simulink model "balancingController_QP"  (Simulink 8.3)
settings: Solver=FixedStepDiscrete  StartTime=0.0  StopTime=inf  FixedStep=Ts  RelTol=1e-3
InitFcn:
  | initBalancingController;
values from neighbouring files (symbols this model uses):
  Gains = block.InputPort(14).Data    [controllerQP.m]    (also in initBalancingController.m = [  120    0   1  1]; initBalancingControllerWithNonLinearImpedances.m = [  70    0   0  4])
  Impedances = block.InputPort(15).Data    [controllerQP.m]    (also in initBalancingController.m = [kImpTorso,kImpArms,kImpArms,kImpLegs,kImpLegs])
undefined symbols (not defined in the file or in its folder): DiscIntNeverNeededParam
undefined symbols (not defined in the file): localName, robotName
libraries: WBCLibrary x18, simulink x2, dspsigops x2
settings Model: Creator=daniele  LastModifiedBy=talha
settings DataIOCC: SignalLoggingSaveFormat=Dataset
settings OptimizationCC: ExpressionDepthLimit=2147483647
settings DebuggingCC: FcnCallInpInsideContextMsg=EnableAllAsWarning
settings SFSimCC: SimParseCustomCode=off

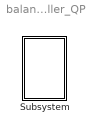
== system balancingController_QP ==
  Subsystem : Subsystem  mask{robotName=robotName, Ts=0.01, localName=localName}
      mask prompts: robotName "robot name"; localName "module name"

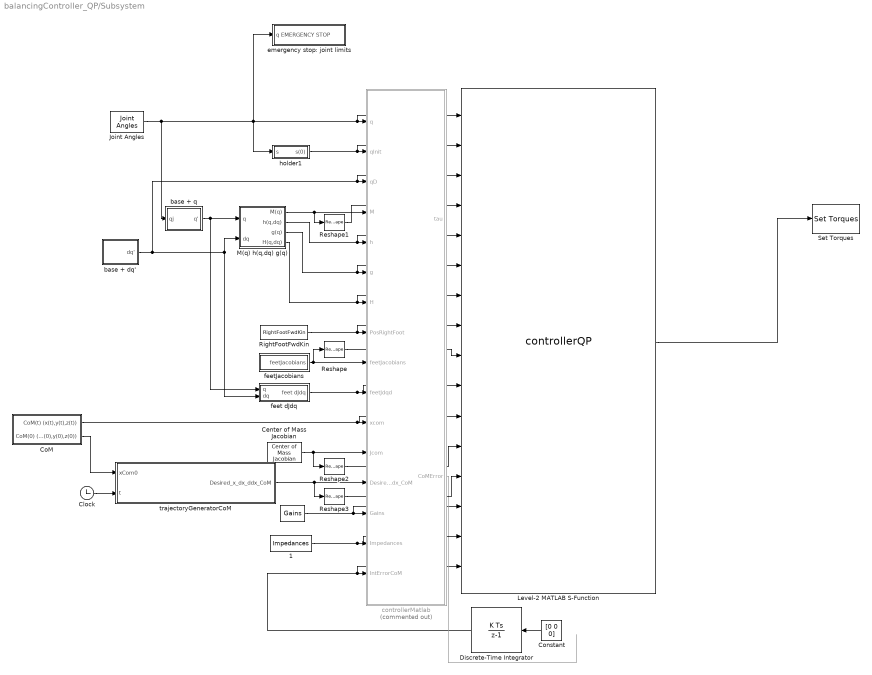
== system balancingController_QP/Subsystem ==
  "    " : Constant  Value=Gains
  "    1" : Constant  Value=Impedances
  Center of Mass Jacobian : WBCLibrary/wholeBodyModel/Jacobians/Center of Mass Jacobian  robotName=robotName  localName=localName
  Clock : Clock
  "CoM " : Subsystem
  Constant : Constant  Value=[0 0 0]
  Discrete-Time Integrator : DiscreteIntegrator  InitialCondition=[0 0 0]  SampleTime=Ts  ICPrevOutput=DiscIntNeverNeededParam  ICPrevScaledInput=DiscIntNeverNeededParam
  Joint Angles : WBCLibrary/wholeBodyStates/Joint Angles  robotName=robotName  localName=localName
  Level-2 MATLAB S-Function : M-S-Function  FunctionName=controllerQP
  M(q) h(q,dq) g(q) : Subsystem
  Reshape{,1..3} (4 alike) : Reshape
  RightFootFwdKin : WBCLibrary/wholeBodyModel/Forward Kinematics/RightFootFwdKin  robotName=robotName  localName=localName
  Set Torques : WBCLibrary/wholeBodyActuators/Set Torques  val=6  robotName=robotName  localName=localName
  base + dq' : Subsystem
  base + q : Subsystem
  controllerMatlab : MATLAB Function  Commented=on  TreatAsAtomicUnit=on
  emergency stop: joint limits : Subsystem
  feet dJdq : Subsystem
  feetJacobians : Subsystem
  holder1 : Subsystem
  trajectoryGeneratorCoM : MATLAB Function  TreatAsAtomicUnit=on
  wires:
  "    "/1 -> controllerMatlab/14(Gains), Level-2 MATLAB S-Function/14
  trajectoryGeneratorCoM/1(Desired_x_dx_ddx_CoM) -> controllerMatlab/13(Desired_x_dx_ddx_CoM), Reshape3/1
  Clock/1 -> trajectoryGeneratorCoM/2(t)
  "CoM "/2(CoM(0) (x(0),y(0),z(0))) -> trajectoryGeneratorCoM/1(xCom0)
  RightFootFwdKin/1 -> Level-2 MATLAB S-Function/8, controllerMatlab/8(PosRightFoot)
  Discrete-Time Integrator/1 -> Level-2 MATLAB S-Function/16, controllerMatlab/16(IntErrorCoM)
  base + q/1(q') -> feet dJdq/1(q), M(q) h(q,dq) g(q)/1(q)
  Joint Angles/1 -> base + q/1(qj), Level-2 MATLAB S-Function/1, controllerMatlab/1(q), emergency stop: joint limits/1(q EMERGENCY STOP), holder1/1(s)
  controllerMatlab/2(CoMError) -> ?
  "    1"/1 -> Level-2 MATLAB S-Function/15, controllerMatlab/15(Impedances)
  M(q) h(q,dq) g(q)/3(g(q)) -> Level-2 MATLAB S-Function/6, controllerMatlab/6(g)
  M(q) h(q,dq) g(q)/4(H(q,dq)) -> Level-2 MATLAB S-Function/7, controllerMatlab/7(H)
  Center of Mass Jacobian/1 -> controllerMatlab/12(Jcom), Reshape2/1
  feetJacobians/1(feetJacobians) -> controllerMatlab/9(feetJacobians), Reshape/1
  feet dJdq/1(feet dJdq) -> Level-2 MATLAB S-Function/10, controllerMatlab/10(feetJdqd)
  holder1/1(s(0)) -> Level-2 MATLAB S-Function/2, controllerMatlab/2(qInit)
  "CoM "/1(CoM(t) (x(t),y(t),z(t))) -> controllerMatlab/11(xcom), Level-2 MATLAB S-Function/11
  base + dq'/1(dq') -> Level-2 MATLAB S-Function/3, controllerMatlab/3(qD), feet dJdq/2(dq), M(q) h(q,dq) g(q)/2(dq)
  M(q) h(q,dq) g(q)/1(M(q)) -> controllerMatlab/4(M), Reshape1/1
  M(q) h(q,dq) g(q)/2(h(q,dq)) -> Level-2 MATLAB S-Function/5, controllerMatlab/5(h)
  Reshape1/1 -> Level-2 MATLAB S-Function/4
  Reshape/1 -> Level-2 MATLAB S-Function/9
  Reshape2/1 -> Level-2 MATLAB S-Function/12
  Reshape3/1 -> Level-2 MATLAB S-Function/13
  Level-2 MATLAB S-Function/1 -> Set Torques/1
  Constant/1 -> Discrete-Time Integrator/1

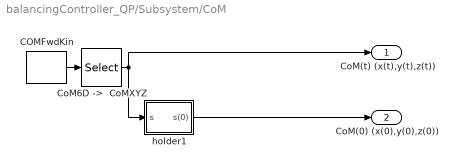
== system balancingController_QP/Subsystem/CoM  ==
  "COMFwdKin " : WBCLibrary/wholeBodyModel/Forward Kinematics/COMFwdKin   robotName=robotName  localName=localName
  "CoM6D ->  CoMXYZ" : Selector  InputPortWidth=7  Indices=[1 2 3]
  holder1 : Subsystem
  CoM(t) (x(t),y(t),z(t)) : Outport
  CoM(0) (x(0),y(0),z(0)) : Outport  Port=2
  wires:
  "COMFwdKin "/1 -> "CoM6D ->  CoMXYZ"/1
  "CoM6D ->  CoMXYZ"/1 -> holder1/1(s), CoM(t) (x(t),y(t),z(t))/1
  holder1/1(s(0)) -> CoM(0) (x(0),y(0),z(0))/1

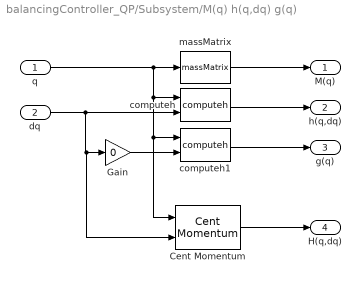
== system balancingController_QP/Subsystem/M(q) h(q,dq) g(q) ==
  q : Inport
  dq : Inport  Port=2
  Cent Momentum : WBCLibrary/wholeBodyModel/Dynamics/Cent Momentum  robotName=robotName  localName=localName
  Gain : Gain  Gain=0
  computeh : WBCLibrary/wholeBodyModel/Dynamics/computeh  val=7  robotname=robotName  localname=localName
  computeh1 : WBCLibrary/wholeBodyModel/Dynamics/computeh  val=7  robotname=robotName  localname=localName
  massMatrix : WBCLibrary/wholeBodyModel/Dynamics/massMatrix  val=8  robotname=robotName  localname=localName
  M(q) : Outport
  h(q,dq) : Outport  Port=2
  g(q) : Outport  Port=3
  H(q,dq) : Outport  Port=4
  wires:
  Gain/1 -> computeh1/2
  computeh1/1 -> g(q)/1
  computeh/1 -> h(q,dq)/1
  massMatrix/1 -> M(q)/1
  q/1 -> Cent Momentum/1, computeh1/1, computeh/1, massMatrix/1
  dq/1 -> Cent Momentum/2, Gain/1, computeh/2
  Cent Momentum/1 -> H(q,dq)/1

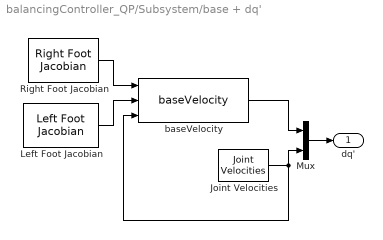
== system balancingController_QP/Subsystem/base + dq' ==
  Joint Velocities : WBCLibrary/wholeBodyStates/Joint Velocities  robotName=robotName  localName=localName
  Left Foot Jacobian : WBCLibrary/wholeBodyModel/Jacobians/Left Foot Jacobian  robotName=robotName  localName=localName
  Mux : Mux  Inputs=2
  Right Foot Jacobian : WBCLibrary/wholeBodyModel/Jacobians/Right Foot Jacobian  robotName=robotName  localName=localName
  baseVelocity : WBCLibrary/Utilities/baseVelocity
  dq' : Outport
  wires:
  Left Foot Jacobian/1 -> baseVelocity/2
  Right Foot Jacobian/1 -> baseVelocity/1
  baseVelocity/1 -> Mux/1
  Joint Velocities/1 -> baseVelocity/3, Mux/2
  Mux/1 -> dq'/1

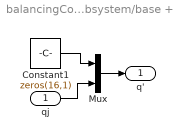
== system balancingController_QP/Subsystem/base + q ==
  qj : Inport
  Constant1 : Constant  Value=zeros(16,1)
  Mux : Mux  Inputs=2
  q' : Outport
  wires:
  Mux/1 -> q'/1
  qj/1 -> Mux/2
  Constant1/1 -> Mux/1

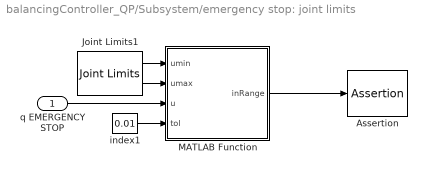
== system balancingController_QP/Subsystem/emergency stop: joint limits ==
  q EMERGENCY STOP : Inport
  Assertion : Assertion
  Joint Limits1 : WBCLibrary/wholeBodyModel/Joint Limits  robotName=robotName  localName=localName
  MATLAB Function : MATLAB Function  TreatAsAtomicUnit=on
  index1 : Constant  Value=0.01  VectorParams1D=off
  wires:
  Joint Limits1/1 -> MATLAB Function/1(umin)
  Joint Limits1/2 -> MATLAB Function/2(umax)
  index1/1 -> MATLAB Function/4(tol)
  q EMERGENCY STOP/1 -> MATLAB Function/3(u)
  MATLAB Function/1(inRange) -> Assertion/1

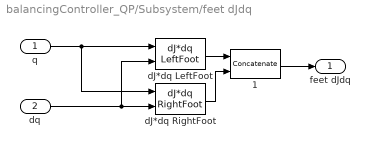
== system balancingController_QP/Subsystem/feet dJdq ==
  q : Inport
  dq : Inport  Port=2
  " 1" : Concatenate  Mode=Multidimensional array
  dJ*dq LeftFoot : WBCLibrary/wholeBodyModel/Dynamics/dJ*dq LeftFoot  val=9  robotName=robotName  localName=localName
  dJ*dq RightFoot : WBCLibrary/wholeBodyModel/Dynamics/dJ*dq RightFoot  val=9  robotName=robotName  localName=localName
  feet dJdq : Outport
  wires:
  dJ*dq LeftFoot/1 -> " 1"/1
  dJ*dq RightFoot/1 -> " 1"/2
  " 1"/1 -> feet dJdq/1
  q/1 -> dJ*dq RightFoot/1, dJ*dq LeftFoot/1
  dq/1 -> dJ*dq LeftFoot/2, dJ*dq RightFoot/2

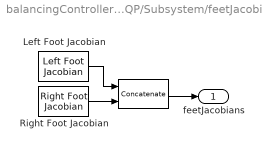
== system balancingController_QP/Subsystem/feetJacobians ==
  " " : Concatenate  Mode=Multidimensional array
  Left Foot Jacobian : WBCLibrary/wholeBodyModel/Jacobians/Left Foot Jacobian  robotName=robotName  localName=localName
  Right Foot Jacobian : WBCLibrary/wholeBodyModel/Jacobians/Right Foot Jacobian  robotName=robotName  localName=localName
  feetJacobians : Outport
  wires:
  Left Foot Jacobian/1 -> " "/1
  Right Foot Jacobian/1 -> " "/2
  " "/1 -> feetJacobians/1

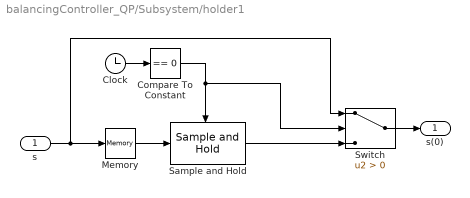
== system balancingController_QP/Subsystem/holder1 ==
  s : Inport
  Clock : Clock
  Compare To Constant : simulink/Logic and Bit Operations/Compare To Constant  relop===  const=0  OutDataTypeStr=boolean
  Memory : Memory
  Sample and Hold : dspsigops/Sample and Hold  trig=Falling edge  initCond=0  latchinput=off
  Switch : Switch  Criteria=u2 > Threshold
  s(0) : Outport
  wires:
  s/1 -> Switch/1, Memory/1
  Clock/1 -> Compare To Constant/1
  Compare To Constant/1 -> Sample and Hold/Trigger, Switch/2
  Sample and Hold/1 -> Switch/3
  Switch/1 -> s(0)/1
  Memory/1 -> Sample and Hold/1

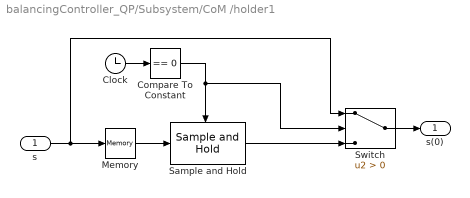
== system balancingController_QP/Subsystem/CoM /holder1 ==
  s : Inport
  Clock : Clock
  Compare To Constant : simulink/Logic and Bit Operations/Compare To Constant  relop===  const=0  OutDataTypeStr=boolean
  Memory : Memory
  Sample and Hold : dspsigops/Sample and Hold  trig=Falling edge  initCond=0  latchinput=off
  Switch : Switch  Criteria=u2 > Threshold
  s(0) : Outport
  wires:
  s/1 -> Switch/1, Memory/1
  Clock/1 -> Compare To Constant/1
  Compare To Constant/1 -> Sample and Hold/Trigger, Switch/2
  Sample and Hold/1 -> Switch/3
  Switch/1 -> s(0)/1
  Memory/1 -> Sample and Hold/1

== matlab function Subsystem/trajectoryGeneratorCoM ==
  data: Desired_x_dx_ddx_CoM output double; xCom0 input double; t input double
function Desired_x_dx_ddx_CoM = fcn(xCom0,t)
%#codegen

e3 = [0;1;0];
A = 0.0;
f = 0.05;

xcomDes    = xCom0 + A*sin(2*pi*f*t)*e3;
% xcomDes(1) =  xcomDes(1) + 0.01;
xDcomDes   =         A*2*pi*f*cos(2*pi*f*t)*e3;
xDDcomDes  =        -A*(2*pi*f)^2*sin(2*pi*f*t)*e3;

Desired_x_dx_ddx_CoM = [xcomDes,xDcomDes,xDDcomDes];

== matlab function Subsystem/controllerMatlab ==
  data: q input double; qInit input double; qD input double; M input double; h input double; g input double; H input double; PosRightFoot input double; feetJacobians input double; tau output double; feetJdqd input double; xcom input double; Jcom input double; Desired_x_dx_ddx_CoM input double; Gains input double; Impedances input double; CoMError output double; IntErrorCoM input double
function [tau,CoMError] = fcn_cont(q,qInit,qD, M, h, g, H, PosRightFoot, feetJacobians, feetJdqd, xcom,Jcom, Desired_x_dx_ddx_CoM, Gains, Impedances, IntErrorCoM)
%#codegen
PINV_TOL = 1e-5;
gravAcc        = 9.81;

n = 25;
St    = [zeros(6,n);eye(n,n)];

m     = M(1,1);
grav = [zeros(2,1);-m*gravAcc;zeros(3,1)];

% Definition of reference accelerations for CoM and Joints that ensure
% stabilization of desired trajectories xDcomDes and qDes 

xDcom      = Jcom(1:3,:)*qD;
xDDcomStar = Desired_x_dx_ddx_CoM(:,3) - Gains(1)*(xcom - Desired_x_dx_ddx_CoM(:,1)) - Gains(2)*IntErrorCoM - Gains(3)*(xDcom - Desired_x_dx_ddx_CoM(:,2));

Pr =  PosRightFoot(1:3) - xcom; % Application point of the contact force on the right foot w.r.t. CoM

A  = [ eye(3),   zeros(3),eye(3), zeros(3);
      -Sf(xcom),  eye(3), Sf(Pr), eye(3) ];
pinvA = pinv(A, PINV_TOL);
  
HDotDes  = [ m*xDDcomStar ;
            -Gains(4)*H(4:end)]; 

Jc    =   feetJacobians;
           
JcDqD = feetJdqd;
            
desiredFeetContactForces = pinvA*(HDotDes-grav);    

Minv = inv(M);
JcMinv        = Jc*Minv;
PInv_JcMinvSt = pinv(JcMinv*St, PINV_TOL);
N0            = eye(n) - PInv_JcMinvSt*JcMinv*St;

measuredFeetContactForces = desiredFeetContactForces;

tauForDesiredFeetForces = PInv_JcMinvSt*(JcMinv*h - JcDqD - JcMinv*Jc'*measuredFeetContactForces);

tauForImpedenceBehaviour = g(7:end)-Jc(:,7:end)'*measuredFeetContactForces - Impedances.*(q-qInit);

tau = tauForDesiredFeetForces + N0*tauForImpedenceBehaviour;

CoMError    = xcom - Desired_x_dx_ddx_CoM(:,1);
normCoMError  = norm(CoMError);




% % function [tau,CoMError] = fcn(q,qInit,qD, M, h, g, H, PosRightFoot, feetJacobians, feetJdqd, xcom,Jcom, Desired_x_dx_ddx_CoM, Gains, Impedances, IntErrorCoM)
% % %#codegen
% % PINV_TOL = 1e-5;
% % gravAcc  = 9.81;
% % 
% % n = 25;
% % St    = [zeros(6,n);eye(n,n)];
% % 
% % m     = M(1,1);
% % Mb    = M(1:6,1:6);
% % Mbj   = M(1:6,7:end);
% % 
% % grav = [zeros(2,1);-m*gravAcc;zeros(3,1)];
% % 
% % % Definition of reference accelerations for CoM and Joints that ensure
% % % stabilization of desired trajectories xDcomDes and qDes 
% % 
% % xDcom      = Jcom(1:3,:)*qD;
% % xDDcomStar = Desired_x_dx_ddx_CoM(:,3) - Gains(1)*(xcom - Desired_x_dx_ddx_CoM(:,1)) - Gains(2)*IntErrorCoM - Gains(3)*(xDcom - Desired_x_dx_ddx_CoM(:,2));
% % 
% % Pr =  PosRightFoot(1:3) - xcom; % Application point of the contact force on the right foot w.r.t. CoM
% % 
% % A  = [ eye(3),   zeros(3),eye(3), zeros(3);
% %       -Sf(xcom),  eye(3), Sf(Pr), eye(3) ];
% % pinvA = pinv(A, PINV_TOL);
% %   
% % HDotDes  = [ m*xDDcomStar ;
% %             -Gains(4)*H(4:end)]; 
% % 
% % Jc    =   feetJacobians;
% %            
% % JcDqD = feetJdqd;
% %             
% % desiredFeetContactForces = pinvA*(HDotDes-grav);    
% % 
% % JcMinv        = Jc/M;
% % PInv_JcMinvSt = pinv(JcMinv*St, PINV_TOL);
% % N0            = eye(n) - PInv_JcMinvSt*JcMinv*St;
% % 
% % measuredFeetContactForces = desiredFeetContactForces;
% % 
% % tauForDesiredFeetForces = PInv_JcMinvSt*(JcMinv*h - JcDqD - JcMinv*Jc'*measuredFeetContactForces);
% % 
% % tauForImpedenceBehaviour = - Impedances.*(q-qInit) + g(7:end)-Jc(:,7:end)'*measuredFeetContactForces - Mbj'/Mb*(h(1:6) - Jc(:,1:6)'*measuredFeetContactForces);
% % 
% % tau = tauForDesiredFeetForces + N0*tauForImpedenceBehaviour;
% % 
% % CoMError    = xcom - Desired_x_dx_ddx_CoM(:,1);
% % % normCoMError  = norm(CoMError);
% % 
% %

== matlab function Subsystem/emergency stop: joint limits/MATLAB Function ==
  data: umin input double; umax input double; u input double; inRange output double; tol input double
function inRange = checkRange(umin, umax, u, tol)
%#codegen

res = u < umin + tol | u > umax - tol;
res = sum(res);
if res==0
    inRange = 1;
else
    inRange = 0;
    u < umin + tol | u > umax - tol
end
